simulink model "final_model"  (Simulink 10.0)
settings: Solver=VariableStepAuto  StartTime=0.0  StopTime=0.1  RelTol=1e-3
model workspace (MAT data in the model file):
  Cth1 = 0.0002995
  Cth2 = 0.0044
  Cth3 = 0.00376
  Irate = 10
  J = 1440
  LM = 0.00639
  Llrp = 0.00824
  Lls = 0.00103
  P = 4
  Psi_ref = 1
  Rd = 1e-05
  Ron = 1e-05
  Rs = 1000000
  Rth1 = 0.085
  Rth2 = 0.353
  Rth3 = 0.7321
  Tref = 15
  Ts = 1e-06
  Vb = 600
  XM = 3.1
  Xlrp = 4
  Xls = 0.5
  battery.e = 200
  battery.r = 1e-05
  battery.c = 0.0002
  battery.cV0 = 100
  load.r = 15
  load.l = 0.2
  m = 0.4
  ref.a = 5
  ref.b = 5
  ref.c = 5
  ref.f = 376.991118431
  rrp = 2.25
  rs = 0.4
  wb = 379
  wt : num (value not decoded)
values from neighbouring files (symbols this model uses):
  Cth1 = 2.995e-4    (= 0.0002995)    [Initialization_naireeta.m]
  Cth2 = 0.0044    [Initialization_naireeta.m]
  Cth3 = 0.00376    [Initialization_naireeta.m]
  Irate = 10    [Initialization_naireeta.m]
  J = 1440    [Initialization_naireeta.m]
  Llrp = 0.00824    [Initialization_naireeta.m]
  Lls = 0.00103    [Initialization_naireeta.m]
  LM = 0.00639    [Initialization_naireeta.m]
  P = 4    [Initialization_naireeta.m]
  rrp = 2.25    [Initialization_naireeta.m]
  rs = 0.4    [Initialization_naireeta.m]
  Rth1 = 0.0850    (= 0.085)    [Initialization_naireeta.m]
  Rth2 = 0.353    [Initialization_naireeta.m]
  Rth3 = 0.7321    [Initialization_naireeta.m]
  Ts = 1e-6    (= 1e-06)    [Initialization_naireeta.m]
libraries: powerlib x135, powerlib_meascontrol x3, simulink x1
(part 1 of 2)
settings Model: Creator=ndeb  LastModifiedBy=ndeb
settings DataIOCC: SaveFormat=Dataset  ReturnWorkspaceOutputs=on
settings OptimizationCC: LifeSpan=auto
settings DebuggingCC: UnderspecifiedInitializationDetection=Simplified  MergeDetectMultiDrivingBlocksExec=error  SFUnexpectedBacktrackingDiag=error  SFNoUnconditionalDefaultTransitionDiag=error  SFExecutionAtInitializationDiag=warning  ArithmeticOperatorsInVariantConditions=error
settings HardwareCC: ProdBitPerPointer=64  ProdBitPerSizeT=64  ProdBitPerPtrDiffT=64  ProdLargestAtomicFloat=Float  ProdIntDivRoundTo=Zero  ProdEndianess=LittleEndian  ProdWordSize=64  ProdHWDeviceType=Intel->x86-64 (Windows64)
settings ModelReferenceCC: PropagateSignalLabelsOutOfModel=on
settings SFSimCC: SimUseLocalCustomCode=on  CustomCodeUndefinedFunction=FilterOut
settings RTWCC: RTWUseLocalCustomCode=on
settings CodeAppCC: StateflowObjectComments=off
settings GRTTargetCC: TargetLangStandard=C99 (ISO)  CombineOutputUpdateFcns=on  GRTInterface=off
settings ConfigComp: CovMetricSettings=dwe  CovHtmlReporting=off  CovSaveCumulativeToWorkspaceVar=off  CovSaveSingleToWorkspaceVar=off

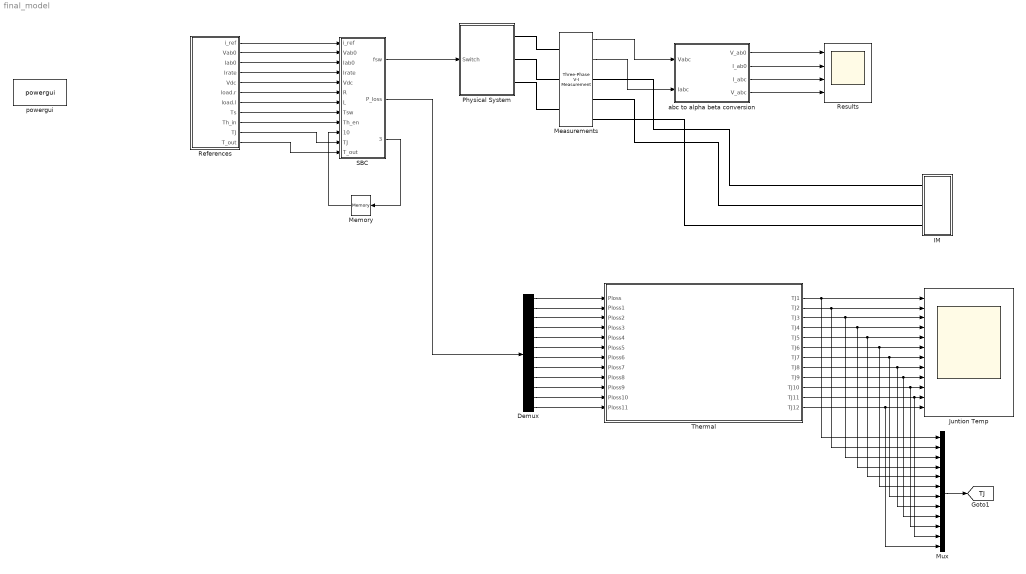
== system final_model ==
  Demux : Demux  Outputs=12
  "IM " : Subsystem
  Juntion Temp : Scope  NumInputPorts=12
  Measurements : powerlib/Measurements/Three-Phase V-I Measurement  VoltageMeasurement=phase-to-ground  SetLabelV=off  LabelV=Vabc  Vpu=off  VpuLL=off  CurrentMeasurement=yes  SetLabelI=off  LabelI=Iabc  Ipu=off  Pbase=100e6  Vbase=500e3  OutputType=Complex  PhasorSimulation=off  PSBequivalent=0
      settings: SourceProductName=Simscape Electrical
  Memory : Memory  InitialCondition=1
  Mux : Mux  Inputs=12
  Physical System : Subsystem
  References : Subsystem
  Results : Scope  NumInputPorts=4
  SBC : MATLAB Function  TreatAsAtomicUnit=on
  "Thermal " : Subsystem
  abc to alpha beta conversion : Subsystem
  powergui : powerlib/powergui  Priority=1  SimulationMode=Discrete  SampleTime=10e-6  frequency=60  Iterations=50  frequencyindice=0  Pbase=100e6  ErrMax=1e-4  UnitsV=kV  UnitsW=MW  buscounter=0  FunctionMessages=off  echomessages=off  EnableUseOfTLC=off  CurrentSourceSwitches=off  DisableSnubberDevices=off  DisableRonSwitches=off  DisableVfSwitches=off  DisplayEquations=off  AutomaticDiscreteSolvers=off  SolverType=Tustin/Backward Euler (TBE)  Interpol=off  ExternalGateDelay=off  methode=off  Ts=100  x0status=blocks  SPID=on  SwTol=0  HookPort=off  NonlinearTolerance=1e-4  nMaxIteration=100  ContinueOnMaxIteration=off  RestoreLinks=warning  ResistiveCurrentMeasurement=off  Frange=[0:2:500]  Ylog=off  Xlog=on  ShowGrid=off  save=off  variable=ZData  structure=0  ZoomFFT=off  StartTime=0.0  cycles=1  DisplayStyle=1  fundamental=60  FreqAxis=off  MaxFrequency=1000  frequencyindicesteady=1  RmsSteady=1  display=off
      settings: SourceProductName=Simscape Electrical
  tag scope: TJ=global
  wires:
  abc to alpha beta conversion/1(V_ab0) -> Results/1
  abc to alpha beta conversion/2("I_ab0 ") -> Results/2
  abc to alpha beta conversion/3(I_abc) -> Results/3
  abc to alpha beta conversion/4(V_abc) -> Results/4
  Measurements/2 -> abc to alpha beta conversion/2(Iabc)
  Measurements/1 -> abc to alpha beta conversion/1(Vabc)
  References/1("i_ref ") -> SBC/1(i_ref)
  References/2(Vab0) -> SBC/2(Vab0)
  References/3(Iab0) -> SBC/3(Iab0)
  References/4("Irate ") -> SBC/4(Irate)
  References/5(Vdc) -> SBC/5(Vdc)
  References/6(load.r) -> SBC/6(R)
  References/7(load.l) -> SBC/7(L)
  References/8(Ts) -> SBC/8(Tsw)
  References/9(Th_in) -> SBC/9(Th_en)
  References/11(T_out) -> SBC/12(T_out)
  SBC/1(fsw) -> Physical System/1("Switch ")
  References/10(TJ) -> SBC/11(TJ)
  SBC/3(Sequence) -> Memory/1
  Memory/1 -> SBC/10(State_p)
  SBC/2(P_loss) -> Demux/1
  Demux/1 -> "Thermal "/1(Ploss)
  Demux/2 -> "Thermal "/2(Ploss1)
  Demux/4 -> "Thermal "/4(Ploss3)
  Demux/3 -> "Thermal "/3(Ploss2)
  Demux/5 -> "Thermal "/5(Ploss4)
  Demux/6 -> "Thermal "/6(Ploss5)
  Demux/7 -> "Thermal "/7(Ploss6)
  Demux/8 -> "Thermal "/8(Ploss7)
  Demux/9 -> "Thermal "/9(Ploss8)
  Demux/10 -> "Thermal "/10(Ploss9)
  Demux/11 -> "Thermal "/11(Ploss10)
  Demux/12 -> "Thermal "/12(Ploss11)
  "Thermal "/1(TJ1) -> Mux/1, Juntion Temp/1
  "Thermal "/2(TJ2) -> Mux/2, Juntion Temp/2
  "Thermal "/3(TJ3) -> Mux/3, Juntion Temp/3
  "Thermal "/4(TJ4) -> Mux/4, Juntion Temp/4
  "Thermal "/5(TJ5) -> Mux/5, Juntion Temp/5
  "Thermal "/6(TJ6) -> Mux/6, Juntion Temp/6
  "Thermal "/7(TJ7) -> Mux/7, Juntion Temp/7
  "Thermal "/8(TJ8) -> Mux/8, Juntion Temp/8
  "Thermal "/9(TJ9) -> Mux/9, Juntion Temp/9
  "Thermal "/10(TJ10) -> Mux/10, Juntion Temp/10
  "Thermal "/11(TJ11) -> Mux/11, Juntion Temp/11
  "Thermal "/12(TJ12) -> Mux/12, Juntion Temp/12
  Mux/1 -> [TJ]
  connections:
  "IM "/LConn1 -- Measurements/RConn1
  Measurements/RConn2 -- "IM "/LConn2
  Measurements/RConn3 -- "IM "/LConn3
  Measurements/LConn1 -- Physical System/RConn1
  Physical System/RConn2 -- Measurements/LConn2
  Physical System/RConn3 -- Measurements/LConn3

== system final_model/IM  ==
  Connection Block : Subsystem
  Dynamic model of IM : Subsystem
  A : PMIOPort  Side=Left
  B : PMIOPort  Port=2  Side=Left
  C : PMIOPort  Port=3  Side=Left
  wires:
  Connection Block/1(Out1) -> Dynamic model of IM/1(a)
  Connection Block/2(Out2) -> Dynamic model of IM/2(b)
  Connection Block/3(Out3) -> Dynamic model of IM/3(c)
  connections:
  Connection Block/LConn3 -- C/RConn1
  Connection Block/LConn1 -- A/RConn1
  Connection Block/LConn2 -- B/RConn1

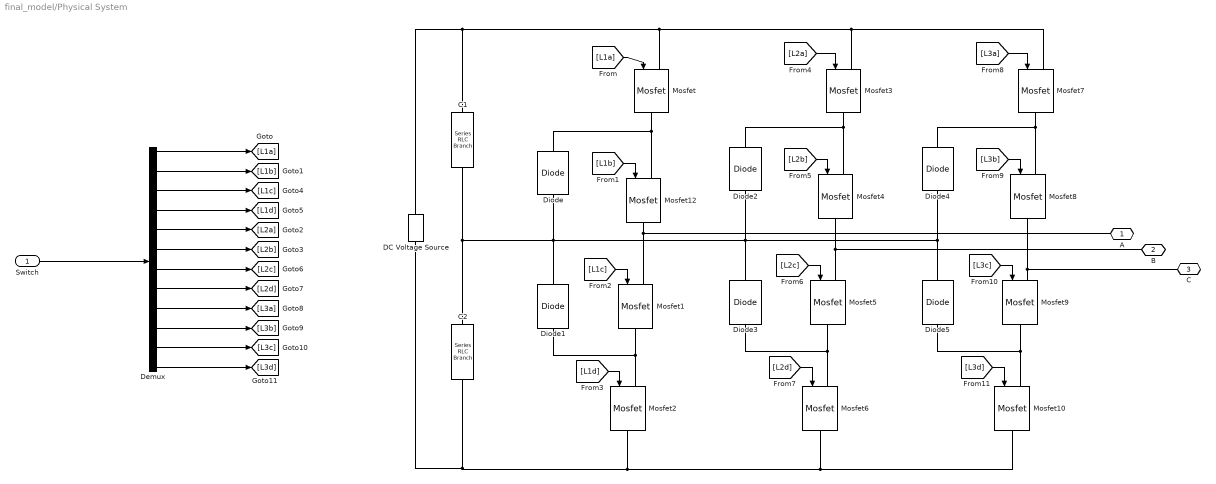
== system final_model/Physical System ==
  "Switch " : Inport
  C1 : powerlib/Elements/Series RLC Branch  LConnTagsString=__new0  RConnTagsString=__new0  BranchType=RC  Resistance=battery.r  Inductance=1.0  SetiL0=off  InitialCurrent=0  Capacitance=battery.c  Setx0=on  InitialVoltage=battery.cV0  Measurements=None
      settings: SourceProductName=Simscape Electrical
  C2 : powerlib/Elements/Series RLC Branch  LConnTagsString=__new0  RConnTagsString=__new0  BranchType=RC  Resistance=battery.r  Inductance=1.0  SetiL0=off  InitialCurrent=0  Capacitance=battery.c  Setx0=on  InitialVoltage=battery.cV0  Measurements=None
      settings: SourceProductName=Simscape Electrical
  DC Voltage Source : powerlib/Electrical Sources/DC Voltage Source  Amplitude=battery.e  Measurements=None
      settings: SourceProductName=Simscape Electrical
  Demux : Demux  Outputs=12
  Diode{,1..5} (6 alike) : powerlib/Power Electronics/Diode  Ron=Ron  Lon=0  Vf=0.8  IC=0  UseSnubber=off  Rs=Rs  Cs=250e-9  Measurements=off
      settings: SourceProductName=Simscape Electrical
  Mosfet{,1..10,12} (12 alike) : powerlib/Power Electronics/Mosfet  Ron=Ron  Lon=0  Rd=Rd  Vfd=0  IC=0  Rs=Rs  Cs=inf  Measurements=off
      settings: SourceProductName=Simscape Electrical
  A : PMIOPort  Side=Right
  B : PMIOPort  Port=2  Side=Right
  C : PMIOPort  Port=3  Side=Right
  wires:
  Demux/7 -> [L2c]
  Demux/4 -> [L1d]
  Demux/3 -> [L1c]
  Demux/5 -> [L2a]
  Demux/8 -> [L2d]
  "Switch "/1 -> Demux/1
  Demux/6 -> [L2b]
  Demux/9 -> [L3a]
  Demux/11 -> [L3c]
  Demux/12 -> [L3d]
  Demux/10 -> [L3b]
  Demux/2 -> [L1b]
  Demux/1 -> [L1a]
  [L1c] -> Mosfet1/1
  [L2a] -> Mosfet3/1
  [L3a] -> Mosfet7/1
  [L3b] -> Mosfet8/1
  [L2b] -> Mosfet4/1
  [L3c] -> Mosfet9/1
  [L1b] -> Mosfet12/1
  [L3d] -> Mosfet10/1
  [L1d] -> Mosfet2/1
  [L2d] -> Mosfet6/1
  [L1a] -> Mosfet/1
  [L2c] -> Mosfet5/1
  connections:
  Diode2/LConn1 -- Diode3/RConn1 -- Diode1/RConn1 -- C1/RConn1 -- C2/LConn1 -- Diode/LConn1 -- Diode5/RConn1 -- Diode4/LConn1
  Mosfet9/LConn1 -- C/RConn1 -- Mosfet8/RConn1
  Mosfet3/LConn1 -- C1/LConn1 -- DC Voltage Source/RConn1 -- Mosfet/LConn1 -- Mosfet7/LConn1
  Mosfet5/RConn1 -- Diode3/LConn1 -- Mosfet6/LConn1
  DC Voltage Source/LConn1 -- Mosfet2/RConn1 -- Mosfet10/RConn1 -- Mosfet6/RConn1 -- C2/RConn1
  Mosfet12/RConn1 -- A/RConn1 -- Mosfet1/LConn1
  Mosfet8/LConn1 -- Diode4/RConn1 -- Mosfet7/RConn1
  Mosfet4/RConn1 -- B/RConn1 -- Mosfet5/LConn1
  Mosfet9/RConn1 -- Diode5/LConn1 -- Mosfet10/LConn1
  Mosfet/RConn1 -- Diode/RConn1 -- Mosfet12/LConn1
  Mosfet4/LConn1 -- Diode2/RConn1 -- Mosfet3/RConn1
  Mosfet1/RConn1 -- Diode1/LConn1 -- Mosfet2/LConn1

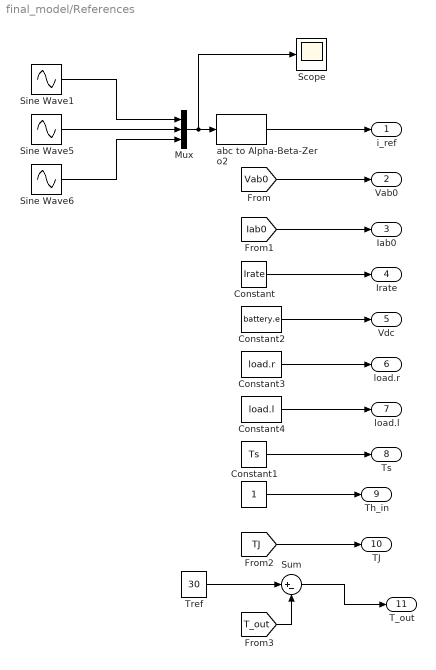
== system final_model/References ==
  " " : Constant  VectorParams1D=off  SampleTime=0
  " Tref" : Constant  Value=30  VectorParams1D=off  SampleTime=0
  Constant : Constant  Value=Irate  VectorParams1D=off  SampleTime=0
  Constant1 : Constant  Value=Ts  VectorParams1D=off  SampleTime=0
  Constant2 : Constant  Value=battery.e  VectorParams1D=off  SampleTime=0
  Constant3 : Constant  Value=load.r  VectorParams1D=off  SampleTime=0
  Constant4 : Constant  Value=load.l  VectorParams1D=off  SampleTime=0
  Mux : Mux  Inputs=3
  Scope : Scope
  Sine Wave1 : Sin  Amplitude=ref.a  Frequency=ref.f  SampleTime=0
  Sine Wave5 : Sin  Amplitude=ref.b  Frequency=ref.f  Phase=-2*pi/3  SampleTime=0
  Sine Wave6 : Sin  Amplitude=ref.c  Frequency=ref.f  Phase=2*pi/3  SampleTime=0
  Sum : Sum  Inputs=|+-
  abc to Alpha-Beta-Zero2 : powerlib_meascontrol/Transformations/abc to Alpha-Beta-Zero
      settings: SourceProductName=Simscape Electrical
  "i_ref " : Outport
  Vab0 : Outport  Port=2
  Iab0 : Outport  Port=3
  "Irate " : Outport  Port=4
  Vdc : Outport  Port=5
  load.r : Outport  Port=6
  load.l : Outport  Port=7
  Ts : Outport  Port=8
  Th_in : Outport  Port=9
  TJ : Outport  Port=10
  T_out : Outport  Port=11
  wires:
  Mux/1 -> Scope/1, abc to Alpha-Beta-Zero2/1
  Sine Wave1/1 -> Mux/1
  abc to Alpha-Beta-Zero2/1 -> "i_ref "/1
  Sine Wave5/1 -> Mux/2
  Constant/1 -> "Irate "/1
  [Vab0] -> Vab0/1
  Sine Wave6/1 -> Mux/3
  [Iab0] -> Iab0/1
  Constant1/1 -> Ts/1
  Constant2/1 -> Vdc/1
  Constant3/1 -> load.r/1
  Constant4/1 -> load.l/1
  " "/1 -> Th_in/1
  [TJ] -> TJ/1
  " Tref"/1 -> Sum/1
  [T_out] -> Sum/2
  Sum/1 -> T_out/1

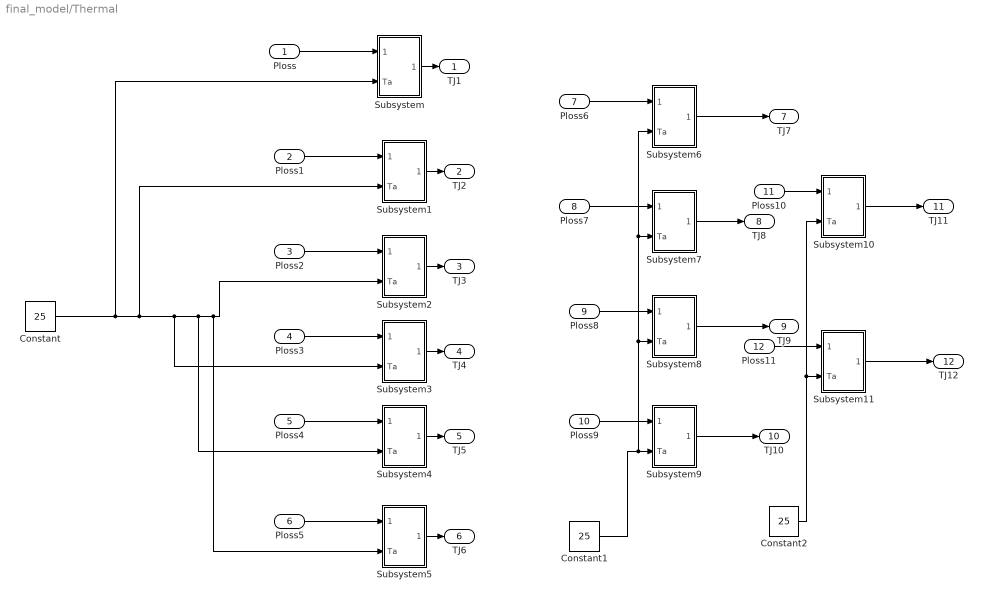
== system final_model/Thermal  ==
  Ploss : Inport
  Ploss1 : Inport  Port=2
  Ploss2 : Inport  Port=3
  Ploss3 : Inport  Port=4
  Ploss4 : Inport  Port=5
  Ploss5 : Inport  Port=6
  Ploss6 : Inport  Port=7
  Ploss7 : Inport  Port=8
  Ploss8 : Inport  Port=9
  Ploss9 : Inport  Port=10
  Ploss10 : Inport  Port=11
  Ploss11 : Inport  Port=12
  Constant : Constant  Value=25
  Constant1 : Constant  Value=25
  Constant2 : Constant  Value=25
  Subsystem : Subsystem
  Subsystem1 : Subsystem
  Subsystem10 : Subsystem
  Subsystem11 : Subsystem
  Subsystem2 : Subsystem
  Subsystem3 : Subsystem
  Subsystem4 : Subsystem
  Subsystem5 : Subsystem
  Subsystem6 : Subsystem
  Subsystem7 : Subsystem
  Subsystem8 : Subsystem
  Subsystem9 : Subsystem
  TJ1 : Outport
  TJ2 : Outport  Port=2
  TJ3 : Outport  Port=3
  TJ4 : Outport  Port=4
  TJ5 : Outport  Port=5
  TJ6 : Outport  Port=6
  TJ7 : Outport  Port=7
  TJ8 : Outport  Port=8
  TJ9 : Outport  Port=9
  TJ10 : Outport  Port=10
  TJ11 : Outport  Port=11
  TJ12 : Outport  Port=12
  wires:
  Subsystem3/1(TJ4) -> TJ4/1
  Ploss/1 -> Subsystem/1(Ploss)
  Constant/1 -> Subsystem/2(Ta), Subsystem1/2(Ta), Subsystem3/2(Ta), Subsystem4/2(Ta), Subsystem5/2(Ta), Subsystem2/2(Ta)
  Subsystem5/1(TJ6) -> TJ6/1
  Ploss3/1 -> Subsystem3/1(Ploss)
  Ploss2/1 -> Subsystem2/1(Ploss)
  Ploss5/1 -> Subsystem5/1(Ploss)
  Ploss1/1 -> Subsystem1/1(Ploss)
  Ploss4/1 -> Subsystem4/1(Ploss)
  Subsystem/1("TJ1 ") -> TJ1/1
  Subsystem2/1(TJ3) -> TJ3/1
  Subsystem4/1(TJ5) -> TJ5/1
  Subsystem1/1(TJ2) -> TJ2/1
  Ploss6/1 -> Subsystem6/1(Ploss)
  Ploss7/1 -> Subsystem7/1(Ploss)
  Ploss8/1 -> Subsystem8/1(Ploss)
  Ploss9/1 -> Subsystem9/1(Ploss)
  Ploss10/1 -> Subsystem10/1(Ploss)
  Ploss11/1 -> Subsystem11/1(Ploss)
  Subsystem6/1("TJ1 ") -> TJ7/1
  Subsystem7/1("TJ1 ") -> TJ8/1
  Subsystem8/1("TJ1 ") -> TJ9/1
  Subsystem9/1("TJ1 ") -> TJ10/1
  Subsystem10/1("TJ1 ") -> TJ11/1
  Subsystem11/1("TJ1 ") -> TJ12/1
  Constant1/1 -> Subsystem6/2(Ta), Subsystem7/2(Ta), Subsystem8/2(Ta), Subsystem9/2(Ta)
  Constant2/1 -> Subsystem10/2(Ta), Subsystem11/2(Ta)

== system final_model/abc to alpha beta conversion ==
  Vabc : Inport
  Iabc : Inport  Port=2
  abc to Alpha-Beta-Zero : powerlib_meascontrol/Transformations/abc to Alpha-Beta-Zero
      settings: SourceProductName=Simscape Electrical
  abc to Alpha-Beta-Zero1 : powerlib_meascontrol/Transformations/abc to Alpha-Beta-Zero
      settings: SourceProductName=Simscape Electrical
  V_ab0 : Outport
  "I_ab0 " : Outport  Port=2
  I_abc : Outport  Port=3
  V_abc : Outport  Port=4
  tag scope: Iab0=global, Vab0=global
  wires:
  Iabc/1 -> I_abc/1, abc to Alpha-Beta-Zero1/1
  abc to Alpha-Beta-Zero/1 -> V_ab0/1, [Vab0]
  Vabc/1 -> V_abc/1, abc to Alpha-Beta-Zero/1
  abc to Alpha-Beta-Zero1/1 -> "I_ab0 "/1, [Iab0]

== system final_model/IM /Connection Block ==
  Ground : powerlib/Elements/Ground  LConnTagsString=a
      settings: SourceProductName=Simscape Electrical
  Voltage Measurement : powerlib/Measurements/Voltage Measurement  PhasorSimulation=off  OutputType=Complex  PSBequivalent=0
      settings: SourceProductName=Simscape Electrical
  Voltage Measurement1 : powerlib/Measurements/Voltage Measurement  PhasorSimulation=off  OutputType=Complex  PSBequivalent=0
      settings: SourceProductName=Simscape Electrical
  Voltage Measurement2 : powerlib/Measurements/Voltage Measurement  PhasorSimulation=off  OutputType=Complex  PSBequivalent=0
      settings: SourceProductName=Simscape Electrical
  Conn1 : PMIOPort  Side=Left
  Conn2 : PMIOPort  Port=2  Side=Left
  Conn3 : PMIOPort  Port=3  Side=Left
  Out1 : Outport
  Out2 : Outport  Port=2
  Out3 : Outport  Port=3
  wires:
  Voltage Measurement1/1 -> Out1/1
  Voltage Measurement/1 -> Out3/1
  Voltage Measurement2/1 -> Out2/1
  connections:
  Voltage Measurement/LConn2 -- Voltage Measurement1/LConn2 -- Voltage Measurement2/LConn2 -- Ground/LConn1
  Voltage Measurement/LConn1 -- Conn3/RConn1
  Voltage Measurement1/LConn1 -- Conn1/RConn1
  Voltage Measurement2/LConn1 -- Conn2/RConn1

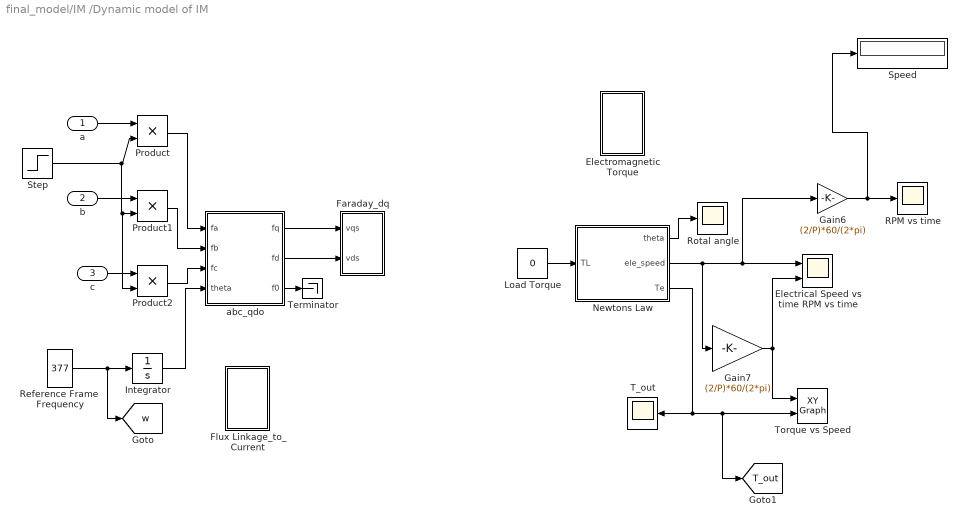
== system final_model/IM /Dynamic model of IM ==
  a : Inport
  b : Inport  Port=2
  c : Inport  Port=3
  Electrical Speed vs time RPM vs time : Scope  NumInputPorts=2
  Electromagnetic Torque : Subsystem
  Faraday_dq : Subsystem
  Flux Linkage_to_Current : Subsystem
  Gain6 : Gain  Gain=(2/P)*60/(2*pi)
  Gain7 : Gain  Gain=(2/P)*60/(2*pi)
  Integrator : Integrator
  Load Torque : Constant  Value=0
  Newtons Law : Subsystem
  Product : Product
  Product1 : Product
  Product2 : Product
  RPM vs time : Scope
  Reference Frame  Frequency : Constant  Value=377
  Rotal angle : Scope
  Speed : Display
  Step : Step  Time=.8  Before=1  After=0  SampleTime=0
  T_out : Scope
  Terminator : Terminator
  Torque vs Speed : simulink/Sinks/XY Graph  xmin=0  xmax=1850  ymin=-25  ymax=125  st=-1
  abc_qdo : Subsystem
  tag scope: T_out=global, w=global
  wires:
  Newtons Law/3(Te) -> [T_out], Torque vs Speed/2, T_out/1
  Newtons Law/2(ele_speed) -> Gain7/1, Electrical Speed vs time RPM vs time/1, Gain6/1
  Gain7/1 -> Torque vs Speed/1, Electrical Speed vs time RPM vs time/2
  Step/1 -> Product2/2, Product1/2, Product/2
  Reference Frame  Frequency/1 -> Integrator/1, [w]
  Newtons Law/1(theta) -> Rotal angle/1
  Gain6/1 -> Speed/1, RPM vs time/1
  Load Torque/1 -> Newtons Law/1(TL)
  abc_qdo/1(fq) -> Faraday_dq/1(vqs)
  a/1 -> Product/1
  Product/1 -> abc_qdo/1(fa)
  Product1/1 -> abc_qdo/2(fb)
  Integrator/1 -> abc_qdo/4(theta)
  abc_qdo/2(fd) -> Faraday_dq/2(vds)
  c/1 -> Product2/1
  b/1 -> Product1/1
  abc_qdo/3(f0) -> Terminator/1
  Product2/1 -> abc_qdo/3(fc)

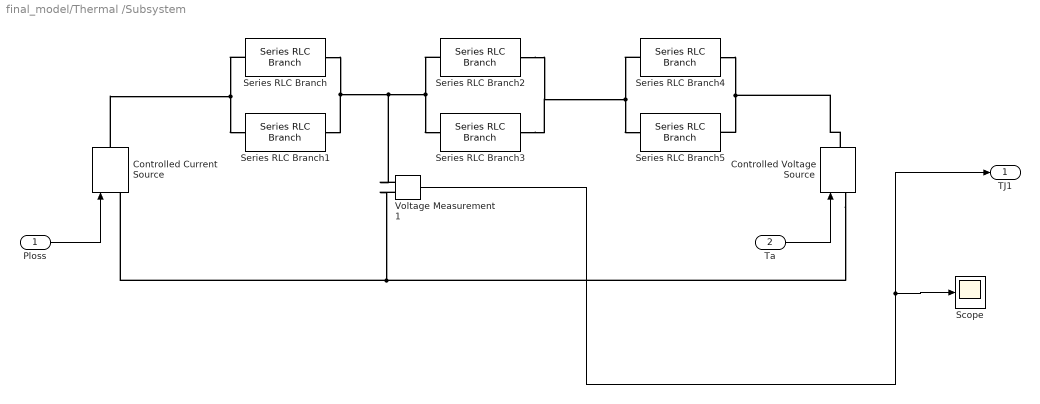
== system final_model/Thermal /Subsystem ==
  Ploss : Inport
  Ta : Inport  Port=2
  Controlled Current Source : powerlib/Electrical Sources/Controlled Current Source  Initialize=on  Source_Type=AC  Amplitude=0  Phase=0  Frequency=0  Measurements=None
      settings: SourceProductName=Simscape Electrical
  Controlled Voltage Source : powerlib/Electrical Sources/Controlled Voltage Source  Initialize=on  Source_Type=AC  Amplitude=0  Phase=0  Frequency=0  Measurements=None
      settings: SourceProductName=Simscape Electrical
  Scope : Scope
  Series RLC Branch : powerlib/Elements/Series RLC Branch  LConnTagsString=__new0  RConnTagsString=__new0  BranchType=R  Resistance=Rth1  Inductance=1e-3  SetiL0=off  InitialCurrent=0  Capacitance=1e-6  Setx0=off  InitialVoltage=0  Measurements=None
      settings: SourceProductName=Simscape Electrical
  Series RLC Branch1 : powerlib/Elements/Series RLC Branch  LConnTagsString=__new0  RConnTagsString=__new0  BranchType=C  Resistance=1  Inductance=1e-3  SetiL0=off  InitialCurrent=0  Capacitance=Cth1  Setx0=off  InitialVoltage=0  Measurements=None
      settings: SourceProductName=Simscape Electrical
  Series RLC Branch2 : powerlib/Elements/Series RLC Branch  LConnTagsString=__new0  RConnTagsString=__new0  BranchType=R  Resistance=Rth2  Inductance=1e-3  SetiL0=off  InitialCurrent=0  Capacitance=1e-6  Setx0=off  InitialVoltage=0  Measurements=None
      settings: SourceProductName=Simscape Electrical
  Series RLC Branch3 : powerlib/Elements/Series RLC Branch  LConnTagsString=__new0  RConnTagsString=__new0  BranchType=C  Resistance=1  Inductance=1e-3  SetiL0=off  InitialCurrent=0  Capacitance=Cth2  Setx0=off  InitialVoltage=0  Measurements=None
      settings: SourceProductName=Simscape Electrical
  Series RLC Branch4 : powerlib/Elements/Series RLC Branch  LConnTagsString=__new0  RConnTagsString=__new0  BranchType=R  Resistance=Rth3  Inductance=1e-3  SetiL0=off  InitialCurrent=0  Capacitance=1e-6  Setx0=off  InitialVoltage=0  Measurements=None
      settings: SourceProductName=Simscape Electrical
  Series RLC Branch5 : powerlib/Elements/Series RLC Branch  LConnTagsString=__new0  RConnTagsString=__new0  BranchType=C  Resistance=1  Inductance=1e-3  SetiL0=off  InitialCurrent=0  Capacitance=Cth3  Setx0=off  InitialVoltage=0  Measurements=None
      settings: SourceProductName=Simscape Electrical
  Voltage Measurement1 : powerlib/Measurements/Voltage Measurement  PhasorSimulation=off  OutputType=Complex  PSBequivalent=0
      settings: SourceProductName=Simscape Electrical
  "TJ1 " : Outport
  wires:
  Ploss/1 -> Controlled Current Source/1
  Ta/1 -> Controlled Voltage Source/1
  Voltage Measurement1/1 -> Scope/1, "TJ1 "/1
  connections:
  Series RLC Branch/LConn1 -- Controlled Current Source/RConn1 -- Series RLC Branch1/LConn1
  Series RLC Branch/RConn1 -- Voltage Measurement1/LConn1 -- Series RLC Branch2/LConn1 -- Series RLC Branch3/LConn1 -- Series RLC Branch1/RConn1
  Controlled Voltage Source/LConn1 -- Voltage Measurement1/LConn2 -- Controlled Current Source/LConn1
  Series RLC Branch4/LConn1 -- Series RLC Branch5/LConn1 -- Series RLC Branch2/RConn1 -- Series RLC Branch3/RConn1
  Series RLC Branch4/RConn1 -- Controlled Voltage Source/RConn1 -- Series RLC Branch5/RConn1

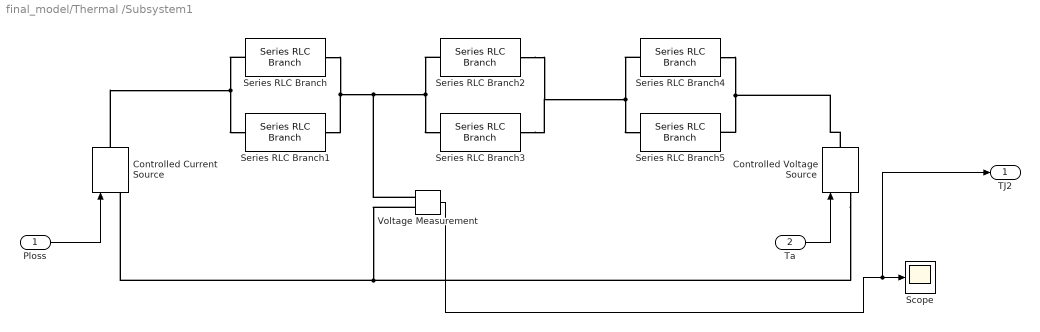
== system final_model/Thermal /Subsystem1 ==
  Ploss : Inport
  Ta : Inport  Port=2
  Controlled Current Source : powerlib/Electrical Sources/Controlled Current Source  Initialize=on  Source_Type=AC  Amplitude=0  Phase=0  Frequency=0  Measurements=None
      settings: SourceProductName=Simscape Electrical
  Controlled Voltage Source : powerlib/Electrical Sources/Controlled Voltage Source  Initialize=on  Source_Type=AC  Amplitude=0  Phase=0  Frequency=0  Measurements=None
      settings: SourceProductName=Simscape Electrical
  Scope : Scope
  Series RLC Branch : powerlib/Elements/Series RLC Branch  LConnTagsString=__new0  RConnTagsString=__new0  BranchType=R  Resistance=Rth1  Inductance=1e-3  SetiL0=off  InitialCurrent=0  Capacitance=1e-6  Setx0=off  InitialVoltage=0  Measurements=None
      settings: SourceProductName=Simscape Electrical
  Series RLC Branch1 : powerlib/Elements/Series RLC Branch  LConnTagsString=__new0  RConnTagsString=__new0  BranchType=C  Resistance=1  Inductance=1e-3  SetiL0=off  InitialCurrent=0  Capacitance=Cth1  Setx0=off  InitialVoltage=0  Measurements=None
      settings: SourceProductName=Simscape Electrical
  Series RLC Branch2 : powerlib/Elements/Series RLC Branch  LConnTagsString=__new0  RConnTagsString=__new0  BranchType=R  Resistance=Rth2  Inductance=1e-3  SetiL0=off  InitialCurrent=0  Capacitance=1e-6  Setx0=off  InitialVoltage=0  Measurements=None
      settings: SourceProductName=Simscape Electrical
  Series RLC Branch3 : powerlib/Elements/Series RLC Branch  LConnTagsString=__new0  RConnTagsString=__new0  BranchType=C  Resistance=1  Inductance=1e-3  SetiL0=off  InitialCurrent=0  Capacitance=Cth2  Setx0=off  InitialVoltage=0  Measurements=None
      settings: SourceProductName=Simscape Electrical
  Series RLC Branch4 : powerlib/Elements/Series RLC Branch  LConnTagsString=__new0  RConnTagsString=__new0  BranchType=R  Resistance=Rth3  Inductance=1e-3  SetiL0=off  InitialCurrent=0  Capacitance=1e-6  Setx0=off  InitialVoltage=0  Measurements=None
      settings: SourceProductName=Simscape Electrical
  Series RLC Branch5 : powerlib/Elements/Series RLC Branch  LConnTagsString=__new0  RConnTagsString=__new0  BranchType=C  Resistance=1  Inductance=1e-3  SetiL0=off  InitialCurrent=0  Capacitance=Cth3  Setx0=off  InitialVoltage=0  Measurements=None
      settings: SourceProductName=Simscape Electrical
  Voltage Measurement : powerlib/Measurements/Voltage Measurement  PhasorSimulation=off  OutputType=Complex  PSBequivalent=0
      settings: SourceProductName=Simscape Electrical
  TJ2 : Outport
  wires:
  Ploss/1 -> Controlled Current Source/1
  Ta/1 -> Controlled Voltage Source/1
  Voltage Measurement/1 -> TJ2/1, Scope/1
  connections:
  Series RLC Branch/LConn1 -- Series RLC Branch1/LConn1 -- Controlled Current Source/RConn1
  Series RLC Branch/RConn1 -- Voltage Measurement/LConn1 -- Series RLC Branch2/LConn1 -- Series RLC Branch3/LConn1 -- Series RLC Branch1/RConn1
  Controlled Voltage Source/LConn1 -- Voltage Measurement/LConn2 -- Controlled Current Source/LConn1
  Series RLC Branch4/LConn1 -- Series RLC Branch5/LConn1 -- Series RLC Branch2/RConn1 -- Series RLC Branch3/RConn1
  Series RLC Branch4/RConn1 -- Controlled Voltage Source/RConn1 -- Series RLC Branch5/RConn1

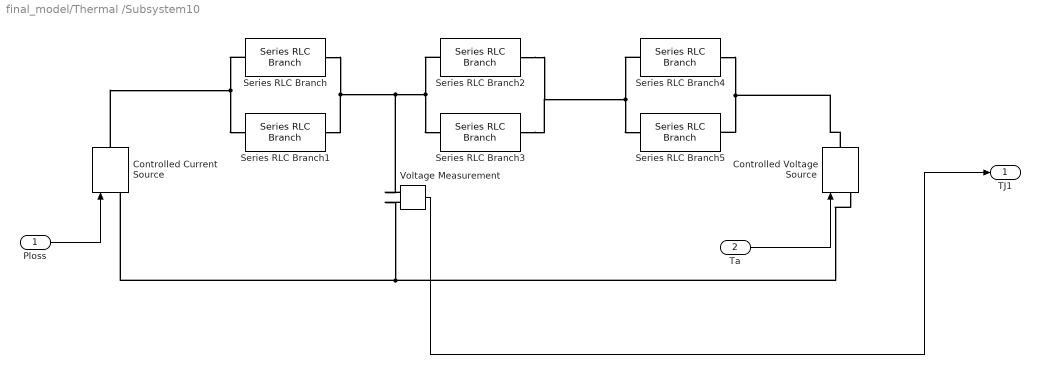
== system final_model/Thermal /Subsystem10 ==
  Ploss : Inport
  Ta : Inport  Port=2
  Controlled Current Source : powerlib/Electrical Sources/Controlled Current Source  Initialize=on  Source_Type=AC  Amplitude=0  Phase=0  Frequency=0  Measurements=None
      settings: SourceProductName=Simscape Electrical
  Controlled Voltage Source : powerlib/Electrical Sources/Controlled Voltage Source  Initialize=on  Source_Type=AC  Amplitude=0  Phase=0  Frequency=0  Measurements=None
      settings: SourceProductName=Simscape Electrical
  Series RLC Branch : powerlib/Elements/Series RLC Branch  LConnTagsString=__new0  RConnTagsString=__new0  BranchType=R  Resistance=Rth1  Inductance=1e-3  SetiL0=off  InitialCurrent=0  Capacitance=1e-6  Setx0=off  InitialVoltage=0  Measurements=None
      settings: SourceProductName=Simscape Electrical
  Series RLC Branch1 : powerlib/Elements/Series RLC Branch  LConnTagsString=__new0  RConnTagsString=__new0  BranchType=C  Resistance=1  Inductance=1e-3  SetiL0=off  InitialCurrent=0  Capacitance=Cth1  Setx0=off  InitialVoltage=0  Measurements=None
      settings: SourceProductName=Simscape Electrical
  Series RLC Branch2 : powerlib/Elements/Series RLC Branch  LConnTagsString=__new0  RConnTagsString=__new0  BranchType=R  Resistance=Rth2  Inductance=1e-3  SetiL0=off  InitialCurrent=0  Capacitance=1e-6  Setx0=off  InitialVoltage=0  Measurements=None
      settings: SourceProductName=Simscape Electrical
  Series RLC Branch3 : powerlib/Elements/Series RLC Branch  LConnTagsString=__new0  RConnTagsString=__new0  BranchType=C  Resistance=1  Inductance=1e-3  SetiL0=off  InitialCurrent=0  Capacitance=Cth2  Setx0=off  InitialVoltage=0  Measurements=None
      settings: SourceProductName=Simscape Electrical
  Series RLC Branch4 : powerlib/Elements/Series RLC Branch  LConnTagsString=__new0  RConnTagsString=__new0  BranchType=R  Resistance=Rth3  Inductance=1e-3  SetiL0=off  InitialCurrent=0  Capacitance=1e-6  Setx0=off  InitialVoltage=0  Measurements=None
      settings: SourceProductName=Simscape Electrical
  Series RLC Branch5 : powerlib/Elements/Series RLC Branch  LConnTagsString=__new0  RConnTagsString=__new0  BranchType=C  Resistance=1  Inductance=1e-3  SetiL0=off  InitialCurrent=0  Capacitance=Cth3  Setx0=off  InitialVoltage=0  Measurements=None
      settings: SourceProductName=Simscape Electrical
  Voltage Measurement : powerlib/Measurements/Voltage Measurement  PhasorSimulation=off  OutputType=Complex  PSBequivalent=0
      settings: SourceProductName=Simscape Electrical
  "TJ1 " : Outport
  wires:
  Ploss/1 -> Controlled Current Source/1
  Ta/1 -> Controlled Voltage Source/1
  Voltage Measurement/1 -> "TJ1 "/1
  connections:
  Series RLC Branch/LConn1 -- Series RLC Branch1/LConn1 -- Controlled Current Source/RConn1
  Series RLC Branch/RConn1 -- Voltage Measurement/LConn1 -- Series RLC Branch2/LConn1 -- Series RLC Branch3/LConn1 -- Series RLC Branch1/RConn1
  Controlled Voltage Source/LConn1 -- Voltage Measurement/LConn2 -- Controlled Current Source/LConn1
  Series RLC Branch4/LConn1 -- Series RLC Branch5/LConn1 -- Series RLC Branch2/RConn1 -- Series RLC Branch3/RConn1
  Series RLC Branch4/RConn1 -- Controlled Voltage Source/RConn1 -- Series RLC Branch5/RConn1

== system final_model/Thermal /Subsystem11 ==
  Ploss : Inport
  Ta : Inport  Port=2
  Controlled Current Source : powerlib/Electrical Sources/Controlled Current Source  Initialize=on  Source_Type=AC  Amplitude=0  Phase=0  Frequency=0  Measurements=None
      settings: SourceProductName=Simscape Electrical
  Controlled Voltage Source : powerlib/Electrical Sources/Controlled Voltage Source  Initialize=on  Source_Type=AC  Amplitude=0  Phase=0  Frequency=0  Measurements=None
      settings: SourceProductName=Simscape Electrical
  Series RLC Branch : powerlib/Elements/Series RLC Branch  LConnTagsString=__new0  RConnTagsString=__new0  BranchType=R  Resistance=Rth1  Inductance=1e-3  SetiL0=off  InitialCurrent=0  Capacitance=1e-6  Setx0=off  InitialVoltage=0  Measurements=None
      settings: SourceProductName=Simscape Electrical
  Series RLC Branch1 : powerlib/Elements/Series RLC Branch  LConnTagsString=__new0  RConnTagsString=__new0  BranchType=C  Resistance=1  Inductance=1e-3  SetiL0=off  InitialCurrent=0  Capacitance=Cth1  Setx0=off  InitialVoltage=0  Measurements=None
      settings: SourceProductName=Simscape Electrical
  Series RLC Branch2 : powerlib/Elements/Series RLC Branch  LConnTagsString=__new0  RConnTagsString=__new0  BranchType=R  Resistance=Rth2  Inductance=1e-3  SetiL0=off  InitialCurrent=0  Capacitance=1e-6  Setx0=off  InitialVoltage=0  Measurements=None
      settings: SourceProductName=Simscape Electrical
  Series RLC Branch3 : powerlib/Elements/Series RLC Branch  LConnTagsString=__new0  RConnTagsString=__new0  BranchType=C  Resistance=1  Inductance=1e-3  SetiL0=off  InitialCurrent=0  Capacitance=Cth2  Setx0=off  InitialVoltage=0  Measurements=None
      settings: SourceProductName=Simscape Electrical
  Series RLC Branch4 : powerlib/Elements/Series RLC Branch  LConnTagsString=__new0  RConnTagsString=__new0  BranchType=R  Resistance=Rth3  Inductance=1e-3  SetiL0=off  InitialCurrent=0  Capacitance=1e-6  Setx0=off  InitialVoltage=0  Measurements=None
      settings: SourceProductName=Simscape Electrical
  Series RLC Branch5 : powerlib/Elements/Series RLC Branch  LConnTagsString=__new0  RConnTagsString=__new0  BranchType=C  Resistance=1  Inductance=1e-3  SetiL0=off  InitialCurrent=0  Capacitance=Cth3  Setx0=off  InitialVoltage=0  Measurements=None
      settings: SourceProductName=Simscape Electrical
  Voltage Measurement : powerlib/Measurements/Voltage Measurement  PhasorSimulation=off  OutputType=Complex  PSBequivalent=0
      settings: SourceProductName=Simscape Electrical
  "TJ1 " : Outport
  wires:
  Ploss/1 -> Controlled Current Source/1
  Ta/1 -> Controlled Voltage Source/1
  Voltage Measurement/1 -> "TJ1 "/1
  connections:
  Series RLC Branch/LConn1 -- Series RLC Branch1/LConn1 -- Controlled Current Source/RConn1
  Series RLC Branch/RConn1 -- Voltage Measurement/LConn1 -- Series RLC Branch2/LConn1 -- Series RLC Branch3/LConn1 -- Series RLC Branch1/RConn1
  Controlled Voltage Source/LConn1 -- Voltage Measurement/LConn2 -- Controlled Current Source/LConn1
  Series RLC Branch4/LConn1 -- Series RLC Branch5/LConn1 -- Series RLC Branch2/RConn1 -- Series RLC Branch3/RConn1
  Series RLC Branch4/RConn1 -- Controlled Voltage Source/RConn1 -- Series RLC Branch5/RConn1

== system final_model/Thermal /Subsystem2 ==
  Ploss : Inport
  Ta : Inport  Port=2
  Controlled Current Source : powerlib/Electrical Sources/Controlled Current Source  Initialize=on  Source_Type=AC  Amplitude=0  Phase=0  Frequency=0  Measurements=None
      settings: SourceProductName=Simscape Electrical
  Controlled Voltage Source : powerlib/Electrical Sources/Controlled Voltage Source  Initialize=on  Source_Type=AC  Amplitude=0  Phase=0  Frequency=0  Measurements=None
      settings: SourceProductName=Simscape Electrical
  Series RLC Branch : powerlib/Elements/Series RLC Branch  LConnTagsString=__new0  RConnTagsString=__new0  BranchType=R  Resistance=Rth1  Inductance=1e-3  SetiL0=off  InitialCurrent=0  Capacitance=1e-6  Setx0=off  InitialVoltage=0  Measurements=None
      settings: SourceProductName=Simscape Electrical
  Series RLC Branch1 : powerlib/Elements/Series RLC Branch  LConnTagsString=__new0  RConnTagsString=__new0  BranchType=C  Resistance=1  Inductance=1e-3  SetiL0=off  InitialCurrent=0  Capacitance=Cth1  Setx0=off  InitialVoltage=0  Measurements=None
      settings: SourceProductName=Simscape Electrical
  Series RLC Branch2 : powerlib/Elements/Series RLC Branch  LConnTagsString=__new0  RConnTagsString=__new0  BranchType=R  Resistance=Rth2  Inductance=1e-3  SetiL0=off  InitialCurrent=0  Capacitance=1e-6  Setx0=off  InitialVoltage=0  Measurements=None
      settings: SourceProductName=Simscape Electrical
  Series RLC Branch3 : powerlib/Elements/Series RLC Branch  LConnTagsString=__new0  RConnTagsString=__new0  BranchType=C  Resistance=1  Inductance=1e-3  SetiL0=off  InitialCurrent=0  Capacitance=Cth2  Setx0=off  InitialVoltage=0  Measurements=None
      settings: SourceProductName=Simscape Electrical
  Series RLC Branch4 : powerlib/Elements/Series RLC Branch  LConnTagsString=__new0  RConnTagsString=__new0  BranchType=R  Resistance=Rth3  Inductance=1e-3  SetiL0=off  InitialCurrent=0  Capacitance=1e-6  Setx0=off  InitialVoltage=0  Measurements=None
      settings: SourceProductName=Simscape Electrical
  Series RLC Branch5 : powerlib/Elements/Series RLC Branch  LConnTagsString=__new0  RConnTagsString=__new0  BranchType=C  Resistance=1  Inductance=1e-3  SetiL0=off  InitialCurrent=0  Capacitance=Cth3  Setx0=off  InitialVoltage=0  Measurements=None
      settings: SourceProductName=Simscape Electrical
  Voltage Measurement : powerlib/Measurements/Voltage Measurement  PhasorSimulation=off  OutputType=Complex  PSBequivalent=0
      settings: SourceProductName=Simscape Electrical
  TJ3 : Outport
  wires:
  Ploss/1 -> Controlled Current Source/1
  Ta/1 -> Controlled Voltage Source/1
  Voltage Measurement/1 -> TJ3/1
  connections:
  Series RLC Branch/LConn1 -- Series RLC Branch1/LConn1 -- Controlled Current Source/RConn1
  Series RLC Branch/RConn1 -- Series RLC Branch2/LConn1 -- Series RLC Branch3/LConn1 -- Voltage Measurement/LConn1 -- Series RLC Branch1/RConn1
  Controlled Voltage Source/LConn1 -- Controlled Current Source/LConn1 -- Voltage Measurement/LConn2
  Series RLC Branch4/LConn1 -- Series RLC Branch5/LConn1 -- Series RLC Branch2/RConn1 -- Series RLC Branch3/RConn1
  Series RLC Branch4/RConn1 -- Controlled Voltage Source/RConn1 -- Series RLC Branch5/RConn1

== system final_model/Thermal /Subsystem3 ==
  Ploss : Inport
  Ta : Inport  Port=2
  Controlled Current Source : powerlib/Electrical Sources/Controlled Current Source  Initialize=on  Source_Type=AC  Amplitude=0  Phase=0  Frequency=0  Measurements=None
      settings: SourceProductName=Simscape Electrical
  Controlled Voltage Source : powerlib/Electrical Sources/Controlled Voltage Source  Initialize=on  Source_Type=AC  Amplitude=0  Phase=0  Frequency=0  Measurements=None
      settings: SourceProductName=Simscape Electrical
  Series RLC Branch : powerlib/Elements/Series RLC Branch  LConnTagsString=__new0  RConnTagsString=__new0  BranchType=R  Resistance=Rth1  Inductance=1e-3  SetiL0=off  InitialCurrent=0  Capacitance=1e-6  Setx0=off  InitialVoltage=0  Measurements=None
      settings: SourceProductName=Simscape Electrical
  Series RLC Branch1 : powerlib/Elements/Series RLC Branch  LConnTagsString=__new0  RConnTagsString=__new0  BranchType=C  Resistance=1  Inductance=1e-3  SetiL0=off  InitialCurrent=0  Capacitance=Cth1  Setx0=off  InitialVoltage=0  Measurements=None
      settings: SourceProductName=Simscape Electrical
  Series RLC Branch2 : powerlib/Elements/Series RLC Branch  LConnTagsString=__new0  RConnTagsString=__new0  BranchType=R  Resistance=Rth2  Inductance=1e-3  SetiL0=off  InitialCurrent=0  Capacitance=1e-6  Setx0=off  InitialVoltage=0  Measurements=None
      settings: SourceProductName=Simscape Electrical
  Series RLC Branch3 : powerlib/Elements/Series RLC Branch  LConnTagsString=__new0  RConnTagsString=__new0  BranchType=C  Resistance=1  Inductance=1e-3  SetiL0=off  InitialCurrent=0  Capacitance=Cth2  Setx0=off  InitialVoltage=0  Measurements=None
      settings: SourceProductName=Simscape Electrical
  Series RLC Branch4 : powerlib/Elements/Series RLC Branch  LConnTagsString=__new0  RConnTagsString=__new0  BranchType=R  Resistance=Rth3  Inductance=1e-3  SetiL0=off  InitialCurrent=0  Capacitance=1e-6  Setx0=off  InitialVoltage=0  Measurements=None
      settings: SourceProductName=Simscape Electrical
  Series RLC Branch5 : powerlib/Elements/Series RLC Branch  LConnTagsString=__new0  RConnTagsString=__new0  BranchType=C  Resistance=1  Inductance=1e-3  SetiL0=off  InitialCurrent=0  Capacitance=Cth3  Setx0=off  InitialVoltage=0  Measurements=None
      settings: SourceProductName=Simscape Electrical
  Voltage Measurement : powerlib/Measurements/Voltage Measurement  PhasorSimulation=off  OutputType=Complex  PSBequivalent=0
      settings: SourceProductName=Simscape Electrical
  TJ4 : Outport
  wires:
  Ploss/1 -> Controlled Current Source/1
  Ta/1 -> Controlled Voltage Source/1
  Voltage Measurement/1 -> TJ4/1
  connections:
  Series RLC Branch/LConn1 -- Series RLC Branch1/LConn1 -- Controlled Current Source/RConn1
  Series RLC Branch/RConn1 -- Series RLC Branch2/LConn1 -- Series RLC Branch3/LConn1 -- Voltage Measurement/LConn1 -- Series RLC Branch1/RConn1
  Controlled Voltage Source/LConn1 -- Voltage Measurement/LConn2 -- Controlled Current Source/LConn1
  Series RLC Branch4/LConn1 -- Series RLC Branch5/LConn1 -- Series RLC Branch2/RConn1 -- Series RLC Branch3/RConn1
  Series RLC Branch4/RConn1 -- Controlled Voltage Source/RConn1 -- Series RLC Branch5/RConn1

== system final_model/Thermal /Subsystem4 ==
  Ploss : Inport
  Ta : Inport  Port=2
  Controlled Current Source : powerlib/Electrical Sources/Controlled Current Source  Initialize=on  Source_Type=AC  Amplitude=0  Phase=0  Frequency=0  Measurements=None
      settings: SourceProductName=Simscape Electrical
  Controlled Voltage Source : powerlib/Electrical Sources/Controlled Voltage Source  Initialize=on  Source_Type=AC  Amplitude=0  Phase=0  Frequency=0  Measurements=None
      settings: SourceProductName=Simscape Electrical
  Series RLC Branch : powerlib/Elements/Series RLC Branch  LConnTagsString=__new0  RConnTagsString=__new0  BranchType=R  Resistance=Rth1  Inductance=1e-3  SetiL0=off  InitialCurrent=0  Capacitance=1e-6  Setx0=off  InitialVoltage=0  Measurements=None
      settings: SourceProductName=Simscape Electrical
  Series RLC Branch1 : powerlib/Elements/Series RLC Branch  LConnTagsString=__new0  RConnTagsString=__new0  BranchType=C  Resistance=1  Inductance=1e-3  SetiL0=off  InitialCurrent=0  Capacitance=Cth1  Setx0=off  InitialVoltage=0  Measurements=None
      settings: SourceProductName=Simscape Electrical
  Series RLC Branch2 : powerlib/Elements/Series RLC Branch  LConnTagsString=__new0  RConnTagsString=__new0  BranchType=R  Resistance=Rth2  Inductance=1e-3  SetiL0=off  InitialCurrent=0  Capacitance=1e-6  Setx0=off  InitialVoltage=0  Measurements=None
      settings: SourceProductName=Simscape Electrical
  Series RLC Branch3 : powerlib/Elements/Series RLC Branch  LConnTagsString=__new0  RConnTagsString=__new0  BranchType=C  Resistance=1  Inductance=1e-3  SetiL0=off  InitialCurrent=0  Capacitance=Cth2  Setx0=off  InitialVoltage=0  Measurements=None
      settings: SourceProductName=Simscape Electrical
  Series RLC Branch4 : powerlib/Elements/Series RLC Branch  LConnTagsString=__new0  RConnTagsString=__new0  BranchType=R  Resistance=Rth3  Inductance=1e-3  SetiL0=off  InitialCurrent=0  Capacitance=1e-6  Setx0=off  InitialVoltage=0  Measurements=None
      settings: SourceProductName=Simscape Electrical
  Series RLC Branch5 : powerlib/Elements/Series RLC Branch  LConnTagsString=__new0  RConnTagsString=__new0  BranchType=C  Resistance=1  Inductance=1e-3  SetiL0=off  InitialCurrent=0  Capacitance=Cth3  Setx0=off  InitialVoltage=0  Measurements=None
      settings: SourceProductName=Simscape Electrical
  Voltage Measurement : powerlib/Measurements/Voltage Measurement  PhasorSimulation=off  OutputType=Complex  PSBequivalent=0
      settings: SourceProductName=Simscape Electrical
  TJ5 : Outport
  wires:
  Ploss/1 -> Controlled Current Source/1
  Ta/1 -> Controlled Voltage Source/1
  Voltage Measurement/1 -> TJ5/1
  connections:
  Series RLC Branch/LConn1 -- Series RLC Branch1/LConn1 -- Controlled Current Source/RConn1
  Series RLC Branch/RConn1 -- Voltage Measurement/LConn1 -- Series RLC Branch2/LConn1 -- Series RLC Branch3/LConn1 -- Series RLC Branch1/RConn1
  Controlled Voltage Source/LConn1 -- Voltage Measurement/LConn2 -- Controlled Current Source/LConn1
  Series RLC Branch4/LConn1 -- Series RLC Branch5/LConn1 -- Series RLC Branch2/RConn1 -- Series RLC Branch3/RConn1
  Series RLC Branch4/RConn1 -- Controlled Voltage Source/RConn1 -- Series RLC Branch5/RConn1

== system final_model/Thermal /Subsystem5 ==
  Ploss : Inport
  Ta : Inport  Port=2
  Controlled Current Source : powerlib/Electrical Sources/Controlled Current Source  Initialize=on  Source_Type=AC  Amplitude=0  Phase=0  Frequency=0  Measurements=None
      settings: SourceProductName=Simscape Electrical
  Controlled Voltage Source : powerlib/Electrical Sources/Controlled Voltage Source  Initialize=on  Source_Type=AC  Amplitude=0  Phase=0  Frequency=0  Measurements=None
      settings: SourceProductName=Simscape Electrical
  Series RLC Branch : powerlib/Elements/Series RLC Branch  LConnTagsString=__new0  RConnTagsString=__new0  BranchType=R  Resistance=Rth1  Inductance=1e-3  SetiL0=off  InitialCurrent=0  Capacitance=1e-6  Setx0=off  InitialVoltage=0  Measurements=None
      settings: SourceProductName=Simscape Electrical
  Series RLC Branch1 : powerlib/Elements/Series RLC Branch  LConnTagsString=__new0  RConnTagsString=__new0  BranchType=C  Resistance=1  Inductance=1e-3  SetiL0=off  InitialCurrent=0  Capacitance=Cth1  Setx0=off  InitialVoltage=0  Measurements=None
      settings: SourceProductName=Simscape Electrical
  Series RLC Branch2 : powerlib/Elements/Series RLC Branch  LConnTagsString=__new0  RConnTagsString=__new0  BranchType=R  Resistance=Rth2  Inductance=1e-3  SetiL0=off  InitialCurrent=0  Capacitance=1e-6  Setx0=off  InitialVoltage=0  Measurements=None
      settings: SourceProductName=Simscape Electrical
  Series RLC Branch3 : powerlib/Elements/Series RLC Branch  LConnTagsString=__new0  RConnTagsString=__new0  BranchType=C  Resistance=1  Inductance=1e-3  SetiL0=off  InitialCurrent=0  Capacitance=Cth2  Setx0=off  InitialVoltage=0  Measurements=None
      settings: SourceProductName=Simscape Electrical
  Series RLC Branch4 : powerlib/Elements/Series RLC Branch  LConnTagsString=__new0  RConnTagsString=__new0  BranchType=R  Resistance=Rth3  Inductance=1e-3  SetiL0=off  InitialCurrent=0  Capacitance=1e-6  Setx0=off  InitialVoltage=0  Measurements=None
      settings: SourceProductName=Simscape Electrical
  Series RLC Branch5 : powerlib/Elements/Series RLC Branch  LConnTagsString=__new0  RConnTagsString=__new0  BranchType=C  Resistance=1  Inductance=1e-3  SetiL0=off  InitialCurrent=0  Capacitance=Cth3  Setx0=off  InitialVoltage=0  Measurements=None
      settings: SourceProductName=Simscape Electrical
  Voltage Measurement : powerlib/Measurements/Voltage Measurement  PhasorSimulation=off  OutputType=Complex  PSBequivalent=0
      settings: SourceProductName=Simscape Electrical
  TJ6 : Outport
  wires:
  Ploss/1 -> Controlled Current Source/1
  Ta/1 -> Controlled Voltage Source/1
  Voltage Measurement/1 -> TJ6/1
  connections:
  Series RLC Branch/LConn1 -- Series RLC Branch1/LConn1 -- Controlled Current Source/RConn1
  Series RLC Branch/RConn1 -- Voltage Measurement/LConn1 -- Series RLC Branch2/LConn1 -- Series RLC Branch3/LConn1 -- Series RLC Branch1/RConn1
  Controlled Voltage Source/LConn1 -- Voltage Measurement/LConn2 -- Controlled Current Source/LConn1
  Series RLC Branch4/LConn1 -- Series RLC Branch5/LConn1 -- Series RLC Branch2/RConn1 -- Series RLC Branch3/RConn1
  Series RLC Branch4/RConn1 -- Controlled Voltage Source/RConn1 -- Series RLC Branch5/RConn1

== system final_model/Thermal /Subsystem6 ==
  Ploss : Inport
  Ta : Inport  Port=2
  Controlled Current Source : powerlib/Electrical Sources/Controlled Current Source  Initialize=on  Source_Type=AC  Amplitude=0  Phase=0  Frequency=0  Measurements=None
      settings: SourceProductName=Simscape Electrical
  Controlled Voltage Source : powerlib/Electrical Sources/Controlled Voltage Source  Initialize=on  Source_Type=AC  Amplitude=0  Phase=0  Frequency=0  Measurements=None
      settings: SourceProductName=Simscape Electrical
  Series RLC Branch : powerlib/Elements/Series RLC Branch  LConnTagsString=__new0  RConnTagsString=__new0  BranchType=R  Resistance=Rth1  Inductance=1e-3  SetiL0=off  InitialCurrent=0  Capacitance=1e-6  Setx0=off  InitialVoltage=0  Measurements=None
      settings: SourceProductName=Simscape Electrical
  Series RLC Branch1 : powerlib/Elements/Series RLC Branch  LConnTagsString=__new0  RConnTagsString=__new0  BranchType=C  Resistance=1  Inductance=1e-3  SetiL0=off  InitialCurrent=0  Capacitance=Cth1  Setx0=off  InitialVoltage=0  Measurements=None
      settings: SourceProductName=Simscape Electrical
  Series RLC Branch2 : powerlib/Elements/Series RLC Branch  LConnTagsString=__new0  RConnTagsString=__new0  BranchType=R  Resistance=Rth2  Inductance=1e-3  SetiL0=off  InitialCurrent=0  Capacitance=1e-6  Setx0=off  InitialVoltage=0  Measurements=None
      settings: SourceProductName=Simscape Electrical
  Series RLC Branch3 : powerlib/Elements/Series RLC Branch  LConnTagsString=__new0  RConnTagsString=__new0  BranchType=C  Resistance=1  Inductance=1e-3  SetiL0=off  InitialCurrent=0  Capacitance=Cth2  Setx0=off  InitialVoltage=0  Measurements=None
      settings: SourceProductName=Simscape Electrical
  Series RLC Branch4 : powerlib/Elements/Series RLC Branch  LConnTagsString=__new0  RConnTagsString=__new0  BranchType=R  Resistance=Rth3  Inductance=1e-3  SetiL0=off  InitialCurrent=0  Capacitance=1e-6  Setx0=off  InitialVoltage=0  Measurements=None
      settings: SourceProductName=Simscape Electrical
  Series RLC Branch5 : powerlib/Elements/Series RLC Branch  LConnTagsString=__new0  RConnTagsString=__new0  BranchType=C  Resistance=1  Inductance=1e-3  SetiL0=off  InitialCurrent=0  Capacitance=Cth3  Setx0=off  InitialVoltage=0  Measurements=None
      settings: SourceProductName=Simscape Electrical
  Voltage Measurement : powerlib/Measurements/Voltage Measurement  PhasorSimulation=off  OutputType=Complex  PSBequivalent=0
      settings: SourceProductName=Simscape Electrical
  "TJ1 " : Outport
  wires:
  Ploss/1 -> Controlled Current Source/1
  Ta/1 -> Controlled Voltage Source/1
  Voltage Measurement/1 -> "TJ1 "/1
  connections:
  Series RLC Branch/LConn1 -- Series RLC Branch1/LConn1 -- Controlled Current Source/RConn1
  Series RLC Branch/RConn1 -- Voltage Measurement/LConn1 -- Series RLC Branch2/LConn1 -- Series RLC Branch3/LConn1 -- Series RLC Branch1/RConn1
  Controlled Voltage Source/LConn1 -- Voltage Measurement/LConn2 -- Controlled Current Source/LConn1
  Series RLC Branch4/LConn1 -- Series RLC Branch5/LConn1 -- Series RLC Branch2/RConn1 -- Series RLC Branch3/RConn1
  Series RLC Branch4/RConn1 -- Controlled Voltage Source/RConn1 -- Series RLC Branch5/RConn1

== system final_model/Thermal /Subsystem7 ==
  Ploss : Inport
  Ta : Inport  Port=2
  Controlled Current Source : powerlib/Electrical Sources/Controlled Current Source  Initialize=on  Source_Type=AC  Amplitude=0  Phase=0  Frequency=0  Measurements=None
      settings: SourceProductName=Simscape Electrical
  Controlled Voltage Source : powerlib/Electrical Sources/Controlled Voltage Source  Initialize=on  Source_Type=AC  Amplitude=0  Phase=0  Frequency=0  Measurements=None
      settings: SourceProductName=Simscape Electrical
  Series RLC Branch : powerlib/Elements/Series RLC Branch  LConnTagsString=__new0  RConnTagsString=__new0  BranchType=R  Resistance=Rth1  Inductance=1e-3  SetiL0=off  InitialCurrent=0  Capacitance=1e-6  Setx0=off  InitialVoltage=0  Measurements=None
      settings: SourceProductName=Simscape Electrical
  Series RLC Branch1 : powerlib/Elements/Series RLC Branch  LConnTagsString=__new0  RConnTagsString=__new0  BranchType=C  Resistance=1  Inductance=1e-3  SetiL0=off  InitialCurrent=0  Capacitance=Cth1  Setx0=off  InitialVoltage=0  Measurements=None
      settings: SourceProductName=Simscape Electrical
  Series RLC Branch2 : powerlib/Elements/Series RLC Branch  LConnTagsString=__new0  RConnTagsString=__new0  BranchType=R  Resistance=Rth2  Inductance=1e-3  SetiL0=off  InitialCurrent=0  Capacitance=1e-6  Setx0=off  InitialVoltage=0  Measurements=None
      settings: SourceProductName=Simscape Electrical
  Series RLC Branch3 : powerlib/Elements/Series RLC Branch  LConnTagsString=__new0  RConnTagsString=__new0  BranchType=C  Resistance=1  Inductance=1e-3  SetiL0=off  InitialCurrent=0  Capacitance=Cth2  Setx0=off  InitialVoltage=0  Measurements=None
      settings: SourceProductName=Simscape Electrical
  Series RLC Branch4 : powerlib/Elements/Series RLC Branch  LConnTagsString=__new0  RConnTagsString=__new0  BranchType=R  Resistance=Rth3  Inductance=1e-3  SetiL0=off  InitialCurrent=0  Capacitance=1e-6  Setx0=off  InitialVoltage=0  Measurements=None
      settings: SourceProductName=Simscape Electrical
  Series RLC Branch5 : powerlib/Elements/Series RLC Branch  LConnTagsString=__new0  RConnTagsString=__new0  BranchType=C  Resistance=1  Inductance=1e-3  SetiL0=off  InitialCurrent=0  Capacitance=Cth3  Setx0=off  InitialVoltage=0  Measurements=None
      settings: SourceProductName=Simscape Electrical
  Voltage Measurement : powerlib/Measurements/Voltage Measurement  PhasorSimulation=off  OutputType=Complex  PSBequivalent=0
      settings: SourceProductName=Simscape Electrical
  "TJ1 " : Outport
  wires:
  Ploss/1 -> Controlled Current Source/1
  Ta/1 -> Controlled Voltage Source/1
  Voltage Measurement/1 -> "TJ1 "/1
  connections:
  Series RLC Branch/LConn1 -- Series RLC Branch1/LConn1 -- Controlled Current Source/RConn1
  Series RLC Branch/RConn1 -- Voltage Measurement/LConn1 -- Series RLC Branch2/LConn1 -- Series RLC Branch3/LConn1 -- Series RLC Branch1/RConn1
  Controlled Voltage Source/LConn1 -- Voltage Measurement/LConn2 -- Controlled Current Source/LConn1
  Series RLC Branch4/LConn1 -- Series RLC Branch5/LConn1 -- Series RLC Branch2/RConn1 -- Series RLC Branch3/RConn1
  Series RLC Branch4/RConn1 -- Controlled Voltage Source/RConn1 -- Series RLC Branch5/RConn1
